simulink model "simulation"  (R2023b)
settings: Solver=VariableStepAuto  StartTime=0.0  StopTime=8  RelTol=1e-3
undefined symbols (not defined in the file or in its folder): intg_z_bap_neg, intg_z_fap_neg, intg_z_iin_neg, intg_z_pzm_neg, intg_z_tus_neg, intg_z_zoh_neg, lead_z_bap_neg, lead_z_fap_neg, lead_z_iin_neg, lead_z_pzm_neg, lead_z_tus_neg, lead_z_zoh_neg
libraries: spsTriangleGeneratorLib x12
settings Model: Creator=camil  LastModifiedBy=camil

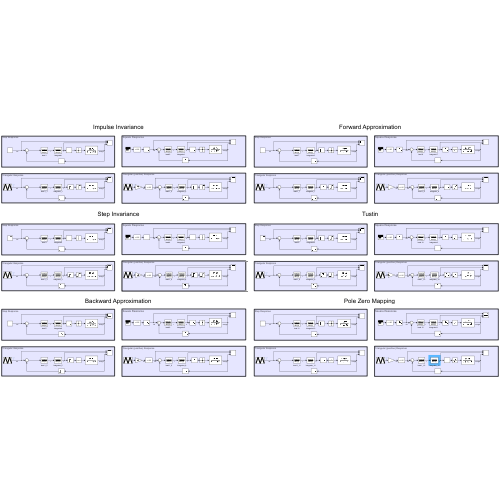
[thumbnail: Simulink's stored preview of the top-level diagram]
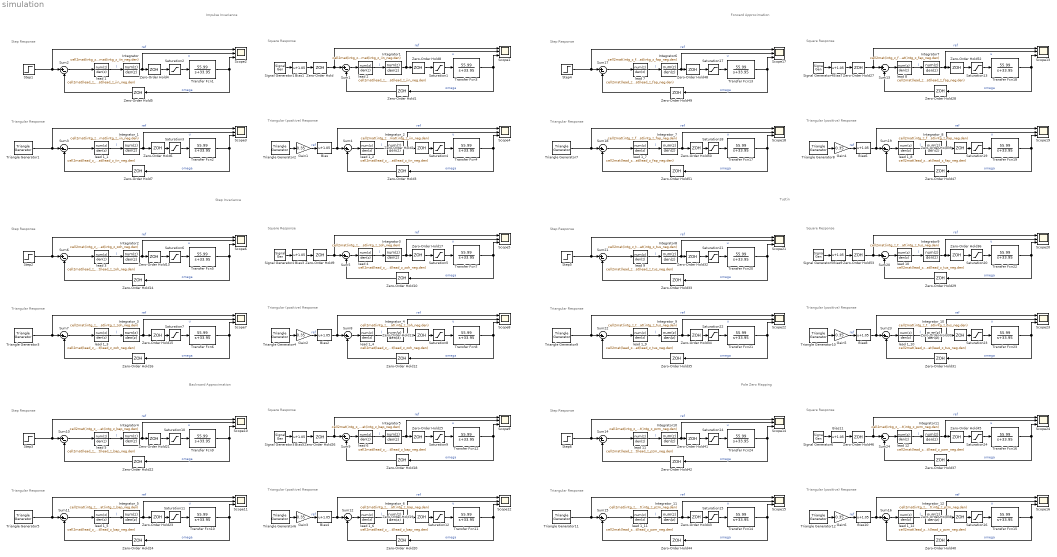
== system simulation ==
  note: Impulse Invariance
  note: Triangular Response
  note: Step Response
  note: Triangular (positive) Response
  note: Square Response
  note: Triangular Response
  note: Triangular (positive) Response
  note: Step Response
  note: Step Invariance
  note: Square Response
  note: Backward Approximation
  note: Square Response
  note: Step Response
  note: Triangular (positive) Response
  note: Triangular Response
  note: Forward Approximation
  note: Triangular (positive) Response
  note: Triangular Response
  note: Step Response
  note: Square Response
  note: Triangular Response
  note: Triangular (positive) Response
  note: Square Response
  note: Tustin
  note: Step Response
  note: Triangular Response
  note: Pole Zero Mapping
  note: Triangular (positive) Response
  note: Step Response
  note: Square Response
  Bias{,1..11} (12 alike) : Bias  Bias=1.05  SaturateOnIntegerOverflow=off
  Gain{1..6} (6 alike) : Gain  Gain=0.35
  Integrator : DiscreteFilter  Numerator=cell2mat(intg_z_iin_neg.num)  Denominator=cell2mat(intg_z_iin_neg.den)
  Integrator1 : DiscreteFilter  Numerator=cell2mat(intg_z_iin_neg.num)  Denominator=cell2mat(intg_z_iin_neg.den)
  Integrator10 : DiscreteFilter  Numerator=cell2mat(intg_z_pzm_neg.num)  Denominator=cell2mat(intg_z_pzm_neg.den)
  Integrator11 : DiscreteFilter  Numerator=cell2mat(intg_z_pzm_neg.num)  Denominator=cell2mat(intg_z_pzm_neg.den)
  Integrator2 : DiscreteFilter  Numerator=cell2mat(intg_z_zoh_neg.num)  Denominator=cell2mat(intg_z_zoh_neg.den)
  Integrator3 : DiscreteFilter  Numerator=cell2mat(intg_z_zoh_neg.num)  Denominator=cell2mat(intg_z_zoh_neg.den)
  Integrator4 : DiscreteFilter  Numerator=cell2mat(intg_z_bap_neg.num)  Denominator=cell2mat(intg_z_bap_neg.den)
  Integrator5 : DiscreteFilter  Numerator=cell2mat(intg_z_bap_neg.num)  Denominator=cell2mat(intg_z_bap_neg.den)
  Integrator6 : DiscreteFilter  Numerator=cell2mat(intg_z_fap_neg.num)  Denominator=cell2mat(intg_z_fap_neg.den)
  Integrator7 : DiscreteFilter  Numerator=cell2mat(intg_z_fap_neg.num)  Denominator=cell2mat(intg_z_fap_neg.den)
  Integrator8 : DiscreteFilter  Numerator=cell2mat(intg_z_tus_neg.num)  Denominator=cell2mat(intg_z_tus_neg.den)
  Integrator9 : DiscreteFilter  Numerator=cell2mat(intg_z_tus_neg.num)  Denominator=cell2mat(intg_z_tus_neg.den)
  Integrator_1 : DiscreteFilter  Numerator=cell2mat(intg_z_iin_neg.num)  Denominator=cell2mat(intg_z_iin_neg.den)
  Integrator_10 : DiscreteFilter  Numerator=cell2mat(intg_z_tus_neg.num)  Denominator=cell2mat(intg_z_tus_neg.den)
  Integrator_11 : DiscreteFilter  Numerator=cell2mat(intg_z_pzm_neg.num)  Denominator=cell2mat(intg_z_pzm_neg.den)
  Integrator_12 : DiscreteFilter  Numerator=cell2mat(intg_z_pzm_neg.num)  Denominator=cell2mat(intg_z_pzm_neg.den)
  Integrator_2 : DiscreteFilter  Numerator=cell2mat(intg_z_iin_neg.num)  Denominator=cell2mat(intg_z_iin_neg.den)
  Integrator_3 : DiscreteFilter  Numerator=cell2mat(intg_z_zoh_neg.num)  Denominator=cell2mat(intg_z_zoh_neg.den)
  Integrator_4 : DiscreteFilter  Numerator=cell2mat(intg_z_zoh_neg.num)  Denominator=cell2mat(intg_z_zoh_neg.den)
  Integrator_5 : DiscreteFilter  Numerator=cell2mat(intg_z_bap_neg.num)  Denominator=cell2mat(intg_z_bap_neg.den)
  Integrator_6 : DiscreteFilter  Numerator=cell2mat(intg_z_bap_neg.num)  Denominator=cell2mat(intg_z_bap_neg.den)
  Integrator_7 : DiscreteFilter  Numerator=cell2mat(intg_z_fap_neg.num)  Denominator=cell2mat(intg_z_fap_neg.den)
  Integrator_8 : DiscreteFilter  Numerator=cell2mat(intg_z_fap_neg.num)  Denominator=cell2mat(intg_z_fap_neg.den)
  Integrator_9 : DiscreteFilter  Numerator=cell2mat(intg_z_tus_neg.num)  Denominator=cell2mat(intg_z_tus_neg.den)
  Saturation{1..24} (24 alike) : Saturate  UpperLimit=1  LowerLimit=-1
  Scope{1..24} (24 alike) : Scope  NumInputPorts=3
  Signal Generator{1..6} (6 alike) : SignalGenerator  WaveForm=square  Amplitude=0.35  Frequency=0.25
  Step{1..6} (6 alike) : Step  SampleTime=0.005
  Sum{1..24} (24 alike) : Sum  Inputs=|+-
  Transfer Fcn{1..24} (24 alike) : TransferFcn  Numerator=[55.99]  Denominator=[1 33.95]
  Triangle Generator{1..12} (12 alike) : spsTriangleGeneratorLib/Triangle Generator  Freq=0.25  Phase=0  Ts=0.005
  Zero-Order Hold{,1..53} (54 alike) : ZeroOrderHold  SampleTime=0.005
  lead 1 : DiscreteFilter  Numerator=cell2mat(lead_z_iin_neg.num)  Denominator=cell2mat(lead_z_iin_neg.den)
  lead 10 : DiscreteFilter  Numerator=cell2mat(lead_z_tus_neg.num)  Denominator=cell2mat(lead_z_tus_neg.den)
  lead 11 : DiscreteFilter  Numerator=cell2mat(lead_z_pzm_neg.num)  Denominator=cell2mat(lead_z_pzm_neg.den)
  lead 12 : DiscreteFilter  Numerator=cell2mat(lead_z_pzm_neg.num)  Denominator=cell2mat(lead_z_pzm_neg.den)
  lead 1_1 : DiscreteFilter  Numerator=cell2mat(lead_z_iin_neg.num)  Denominator=cell2mat(lead_z_iin_neg.den)
  lead 1_10 : DiscreteFilter  Numerator=cell2mat(lead_z_tus_neg.num)  Denominator=cell2mat(lead_z_tus_neg.den)
  lead 1_11 : DiscreteFilter  Numerator=cell2mat(lead_z_pzm_neg.num)  Denominator=cell2mat(lead_z_pzm_neg.den)
  lead 1_12 : DiscreteFilter  Numerator=cell2mat(lead_z_pzm_neg.num)  Denominator=cell2mat(lead_z_pzm_neg.den)
  lead 1_2 : DiscreteFilter  Numerator=cell2mat(lead_z_iin_neg.num)  Denominator=cell2mat(lead_z_iin_neg.den)
  lead 1_3 : DiscreteFilter  Numerator=cell2mat(lead_z_zoh_neg.num)  Denominator=cell2mat(lead_z_zoh_neg.den)
  lead 1_4 : DiscreteFilter  Numerator=cell2mat(lead_z_zoh_neg.num)  Denominator=cell2mat(lead_z_zoh_neg.den)
  lead 1_5 : DiscreteFilter  Numerator=cell2mat(lead_z_bap_neg.num)  Denominator=cell2mat(lead_z_bap_neg.den)
  lead 1_6 : DiscreteFilter  Numerator=cell2mat(lead_z_bap_neg.num)  Denominator=cell2mat(lead_z_bap_neg.den)
  lead 1_7 : DiscreteFilter  Numerator=cell2mat(lead_z_fap_neg.num)  Denominator=cell2mat(lead_z_fap_neg.den)
  lead 1_8 : DiscreteFilter  Numerator=cell2mat(lead_z_fap_neg.num)  Denominator=cell2mat(lead_z_fap_neg.den)
  lead 1_9 : DiscreteFilter  Numerator=cell2mat(lead_z_tus_neg.num)  Denominator=cell2mat(lead_z_tus_neg.den)
  lead 2 : DiscreteFilter  Numerator=cell2mat(lead_z_iin_neg.num)  Denominator=cell2mat(lead_z_iin_neg.den)
  lead 3 : DiscreteFilter  Numerator=cell2mat(lead_z_zoh_neg.num)  Denominator=cell2mat(lead_z_zoh_neg.den)
  lead 4 : DiscreteFilter  Numerator=cell2mat(lead_z_zoh_neg.num)  Denominator=cell2mat(lead_z_zoh_neg.den)
  lead 5 : DiscreteFilter  Numerator=cell2mat(lead_z_bap_neg.num)  Denominator=cell2mat(lead_z_bap_neg.den)
  lead 6 : DiscreteFilter  Numerator=cell2mat(lead_z_bap_neg.num)  Denominator=cell2mat(lead_z_bap_neg.den)
  lead 7 : DiscreteFilter  Numerator=cell2mat(lead_z_fap_neg.num)  Denominator=cell2mat(lead_z_fap_neg.den)
  lead 8 : DiscreteFilter  Numerator=cell2mat(lead_z_fap_neg.num)  Denominator=cell2mat(lead_z_fap_neg.den)
  lead 9 : DiscreteFilter  Numerator=cell2mat(lead_z_tus_neg.num)  Denominator=cell2mat(lead_z_tus_neg.den)
  wires:
  Saturation2/1 -> Transfer Fcn1/1
  Zero-Order Hold4/1 -> Saturation2/1
  Step1/1 -> Sum2/1, Scope2/1  "ref"
  Zero-Order Hold5/1 -> Sum2/2
  Transfer Fcn1/1 -> Scope2/3, Zero-Order Hold5/1  "omega"
  Sum2/1 -> lead 1/1
  lead 1/1 -> Integrator/1  "l"
  Integrator/1 -> Scope2/2, Zero-Order Hold4/1  "u"
  Zero-Order Hold7/1 -> Sum3/2
  lead 1_1/1 -> Integrator_1/1  "l"
  Integrator_1/1 -> Zero-Order Hold6/1, Scope3/2  "u"
  Zero-Order Hold6/1 -> Saturation3/1
  Sum3/1 -> lead 1_1/1
  Triangle Generator1/1 -> Sum3/1, Scope3/1  "ref"
  Saturation3/1 -> Transfer Fcn2/1
  Transfer Fcn2/1 -> Scope3/3, Zero-Order Hold7/1  "omega"
  Sum4/1 -> lead 1_2/1
  Zero-Order Hold3/1 -> Sum4/2
  Transfer Fcn4/1 -> Scope4/3, Zero-Order Hold3/1  "omega"
  Saturation4/1 -> Transfer Fcn4/1
  lead 1_2/1 -> Integrator_2/1  "l"
  Sum1/1 -> lead 2/1
  Transfer Fcn3/1 -> Scope1/3, Zero-Order Hold1/1  "omega"
  Bias1/1 -> Zero-Order Hold/1
  Integrator_2/1 -> Zero-Order Hold2/1, Scope4/2  "u"
  Zero-Order Hold2/1 -> Saturation4/1
  Integrator1/1 -> Scope1/2, Zero-Order Hold8/1  "u"
  Zero-Order Hold8/1 -> Saturation1/1
  Saturation1/1 -> Transfer Fcn3/1
  Zero-Order Hold1/1 -> Sum1/2
  lead 2/1 -> Integrator1/1  "l"
  Bias/1 -> Scope4/1, Sum4/1  "ref"
  Triangle Generator2/1 -> Gain1/1
  Gain1/1 -> Bias/1  "ref"
  Signal Generator1/1 -> Bias1/1
  Zero-Order Hold/1 -> Scope1/1, Sum1/1  "ref"
  Transfer Fcn7/1 -> Scope5/3, Zero-Order Hold10/1  "omega"
  Integrator_3/1 -> Zero-Order Hold15/1, Scope7/2  "u"
  Zero-Order Hold11/1 -> Saturation8/1
  Saturation5/1 -> Transfer Fcn7/1
  Transfer Fcn6/1 -> Scope7/3, Zero-Order Hold16/1  "omega"
  lead 3/1 -> Integrator2/1  "l"
  Integrator2/1 -> Scope6/2, Zero-Order Hold13/1  "u"
  Sum8/1 -> lead 1_4/1
  Zero-Order Hold9/1 -> Scope5/1, Sum5/1  "ref"
  Saturation7/1 -> Transfer Fcn6/1
  Saturation8/1 -> Transfer Fcn8/1
  Transfer Fcn8/1 -> Scope8/3, Zero-Order Hold12/1  "omega"
  Zero-Order Hold12/1 -> Sum8/2
  Triangle Generator3/1 -> Sum7/1, Scope7/1  "ref"
  Sum5/1 -> lead 4/1
  Step2/1 -> Sum6/1, Scope6/1  "ref"
  Bias2/1 -> Scope8/1, Sum8/1  "ref"
  Saturation6/1 -> Transfer Fcn5/1
  Sum7/1 -> lead 1_3/1
  Zero-Order Hold15/1 -> Saturation7/1
  Zero-Order Hold16/1 -> Sum7/2
  lead 1_3/1 -> Integrator_3/1  "l"
  Zero-Order Hold10/1 -> Sum5/2
  lead 4/1 -> Integrator3/1  "l"
  Bias3/1 -> Zero-Order Hold9/1
  Signal Generator2/1 -> Bias3/1
  Gain2/1 -> Bias2/1  "ref"
  lead 1_4/1 -> Integrator_4/1  "l"
  Sum6/1 -> lead 3/1
  Zero-Order Hold13/1 -> Saturation6/1
  Integrator3/1 -> Scope5/2, Zero-Order Hold17/1  "u"
  Triangle Generator4/1 -> Gain2/1
  Integrator_4/1 -> Zero-Order Hold11/1, Scope8/2  "u"
  Transfer Fcn5/1 -> Scope6/3, Zero-Order Hold14/1  "omega"
  Zero-Order Hold17/1 -> Saturation5/1
  Zero-Order Hold14/1 -> Sum6/2
  Transfer Fcn10/1 -> Scope11/3, Zero-Order Hold24/1  "omega"
  Integrator_5/1 -> Zero-Order Hold23/1, Scope11/2  "u"
  Zero-Order Hold19/1 -> Saturation12/1
  Saturation9/1 -> Transfer Fcn12/1
  Transfer Fcn12/1 -> Scope9/3, Zero-Order Hold18/1  "omega"
  Sum9/1 -> lead 6/1
  Bias4/1 -> Scope12/1, Sum12/1  "ref"
  lead 5/1 -> Integrator4/1  "l"
  Triangle Generator5/1 -> Sum11/1, Scope11/1  "ref"
  Transfer Fcn11/1 -> Scope12/3, Zero-Order Hold20/1  "omega"
  Step3/1 -> Sum10/1, Scope10/1  "ref"
  Saturation11/1 -> Transfer Fcn10/1
  Saturation12/1 -> Transfer Fcn11/1
  Zero-Order Hold26/1 -> Scope9/1, Sum9/1  "ref"
  Integrator4/1 -> Scope10/2, Zero-Order Hold21/1  "u"
  Zero-Order Hold21/1 -> Saturation10/1
  Integrator5/1 -> Scope9/2, Zero-Order Hold25/1  "u"
  lead 1_6/1 -> Integrator_6/1  "l"
  Gain3/1 -> Bias4/1  "ref"
  Bias5/1 -> Zero-Order Hold26/1
  Triangle Generator6/1 -> Gain3/1
  Signal Generator3/1 -> Bias5/1
  lead 1_5/1 -> Integrator_5/1  "l"
  Zero-Order Hold20/1 -> Sum12/2
  Saturation10/1 -> Transfer Fcn9/1
  lead 6/1 -> Integrator5/1  "l"
  Zero-Order Hold24/1 -> Sum11/2
  Integrator_6/1 -> Zero-Order Hold19/1, Scope12/2  "u"
  Zero-Order Hold18/1 -> Sum9/2
  Sum12/1 -> lead 1_6/1
  Zero-Order Hold23/1 -> Saturation11/1
  Sum10/1 -> lead 5/1
  Zero-Order Hold25/1 -> Saturation9/1
  Zero-Order Hold22/1 -> Sum10/2
  Transfer Fcn9/1 -> Scope10/3, Zero-Order Hold22/1  "omega"
  Sum11/1 -> lead 1_5/1
  Saturation22/1 -> Transfer Fcn21/1
  Transfer Fcn21/1 -> Scope22/3, Zero-Order Hold35/1  "omega"
  Zero-Order Hold42/1 -> Sum14/2
  Bias11/1 -> Zero-Order Hold46/1
  Sum15/1 -> lead 1_11/1
  Triangle Generator11/1 -> Sum15/1, Scope15/1  "ref"
  Integrator_7/1 -> Zero-Order Hold50/1, Scope18/2  "u"
  Zero-Order Hold45/1 -> Saturation24/1
  Sum14/1 -> lead 11/1
  Zero-Order Hold53/1 -> Scope20/1, Sum20/1  "ref"
  Bias10/1 -> Scope16/1, Sum16/1  "ref"
  Zero-Order Hold43/1 -> Saturation15/1
  lead 12/1 -> Integrator11/1  "l"
  Zero-Order Hold37/1 -> Sum24/2
  Integrator6/1 -> Scope17/2, Zero-Order Hold48/1  "u"
  Zero-Order Hold49/1 -> Sum17/2
  lead 1_11/1 -> Integrator_11/1  "l"
  Gain6/1 -> Bias10/1  "ref"
  Zero-Order Hold40/1 -> Sum16/2
  Signal Generator6/1 -> Bias11/1
  lead 1_9/1 -> Integrator_9/1  "l"
  Zero-Order Hold44/1 -> Sum15/2
  Bias8/1 -> Scope23/1, Sum23/1  "ref"
  Sum16/1 -> lead 1_12/1
  Sum21/1 -> lead 9/1
  Integrator_8/1 -> Zero-Order Hold39/1, Scope19/2  "u"
  lead 11/1 -> Integrator10/1  "l"
  Zero-Order Hold38/1 -> Saturation16/1
  Integrator11/1 -> Scope24/2, Zero-Order Hold45/1  "u"
  Zero-Order Hold41/1 -> Saturation14/1
  Integrator10/1 -> Scope14/2, Zero-Order Hold41/1  "u"
  Zero-Order Hold29/1 -> Sum20/2
  Triangle Generator12/1 -> Gain6/1
  Sum18/1 -> lead 1_7/1
  Step6/1 -> Sum14/1, Scope14/1  "ref"
  Bias9/1 -> Zero-Order Hold53/1
  Triangle Generator10/1 -> Gain5/1
  Zero-Order Hold46/1 -> Scope24/1, Sum24/1  "ref"
  lead 1_8/1 -> Integrator_8/1  "l"
  Zero-Order Hold51/1 -> Sum18/2
  Integrator9/1 -> Scope20/2, Zero-Order Hold36/1  "u"
  Zero-Order Hold33/1 -> Sum21/2
  Zero-Order Hold32/1 -> Saturation21/1
  Step5/1 -> Sum21/1, Scope21/1  "ref"
  Zero-Order Hold36/1 -> Saturation20/1
  Integrator_10/1 -> Zero-Order Hold30/1, Scope23/2  "u"
  Zero-Order Hold31/1 -> Sum23/2
  Sum20/1 -> lead 10/1
  Zero-Order Hold27/1 -> Scope13/1, Sum13/1  "ref"
  lead 10/1 -> Integrator9/1  "l"
  Sum23/1 -> lead 1_10/1
  Sum22/1 -> lead 1_9/1
  Gain5/1 -> Bias8/1  "ref"
  Sum19/1 -> lead 1_8/1
  Zero-Order Hold34/1 -> Saturation22/1
  Signal Generator5/1 -> Bias9/1
  lead 1_12/1 -> Integrator_12/1  "l"
  Zero-Order Hold35/1 -> Sum22/2
  Zero-Order Hold48/1 -> Saturation17/1
  lead 9/1 -> Integrator8/1  "l"
  Triangle Generator9/1 -> Sum22/1, Scope22/1  "ref"
  Triangle Generator8/1 -> Gain4/1
  Bias6/1 -> Scope19/1, Sum19/1  "ref"
  lead 8/1 -> Integrator7/1  "l"
  Gain4/1 -> Bias6/1  "ref"
  Zero-Order Hold30/1 -> Saturation23/1
  Triangle Generator7/1 -> Sum18/1, Scope18/1  "ref"
  Step4/1 -> Sum17/1, Scope17/1  "ref"
  Sum13/1 -> lead 8/1
  Sum24/1 -> lead 12/1
  Zero-Order Hold50/1 -> Saturation18/1
  Zero-Order Hold47/1 -> Sum19/2
  Bias7/1 -> Zero-Order Hold27/1
  Zero-Order Hold28/1 -> Sum13/2
  Integrator7/1 -> Scope13/2, Zero-Order Hold52/1  "u"
  Integrator_11/1 -> Zero-Order Hold43/1, Scope15/2  "u"
  Sum17/1 -> lead 7/1
  Signal Generator4/1 -> Bias7/1
  lead 7/1 -> Integrator6/1  "l"
  lead 1_7/1 -> Integrator_7/1  "l"
  Saturation14/1 -> Transfer Fcn24/1
  Transfer Fcn24/1 -> Scope14/3, Zero-Order Hold42/1  "omega"
  Integrator8/1 -> Scope21/2, Zero-Order Hold32/1  "u"
  Saturation21/1 -> Transfer Fcn20/1
  Integrator_9/1 -> Zero-Order Hold34/1, Scope22/2  "u"
  Transfer Fcn20/1 -> Scope21/3, Zero-Order Hold33/1  "omega"
  lead 1_10/1 -> Integrator_10/1  "l"
  Transfer Fcn13/1 -> Scope17/3, Zero-Order Hold49/1  "omega"
  Saturation17/1 -> Transfer Fcn13/1
  Saturation19/1 -> Transfer Fcn19/1
  Transfer Fcn22/1 -> Scope20/3, Zero-Order Hold29/1  "omega"
  Saturation24/1 -> Transfer Fcn16/1
  Zero-Order Hold39/1 -> Saturation19/1
  Transfer Fcn16/1 -> Scope24/3, Zero-Order Hold37/1  "omega"
  Saturation13/1 -> Transfer Fcn18/1
  Zero-Order Hold52/1 -> Saturation13/1
  Transfer Fcn18/1 -> Scope13/3, Zero-Order Hold28/1  "omega"
  Transfer Fcn23/1 -> Scope23/3, Zero-Order Hold31/1  "omega"
  Saturation23/1 -> Transfer Fcn23/1
  Saturation16/1 -> Transfer Fcn15/1
  Transfer Fcn19/1 -> Scope19/3, Zero-Order Hold47/1  "omega"
  Transfer Fcn15/1 -> Scope16/3, Zero-Order Hold40/1  "omega"
  Saturation18/1 -> Transfer Fcn17/1
  Transfer Fcn17/1 -> Scope18/3, Zero-Order Hold51/1  "omega"
  Transfer Fcn14/1 -> Scope15/3, Zero-Order Hold44/1  "omega"
  Saturation20/1 -> Transfer Fcn22/1
  Saturation15/1 -> Transfer Fcn14/1
  Integrator_12/1 -> Zero-Order Hold38/1, Scope16/2  "u"
